simulink model "Buck_Boost_converter_Lab"  (R2020b)
settings: Solver=ode23tb  StartTime=0.0  StopTime=1  RelTol=1e-3
values from neighbouring files (symbols this model uses):
  C = 2200e-6    (= 0.0022)    [Parameters.m]    (also in Parameters_Buck_Boost.m = 0.00022; boost.m = 0.00022)
  d = 0.5    [Parameters.m]    (also in Parameters_Buck_Boost.m; boost.m)
  f = 5000    [Parameters.m]    (also in Parameters_Buck_Boost.m; boost.m)
  L = 820e-6    (= 0.00082)    [Parameters.m]    (also in Parameters_Buck_Boost.m = 0.0008; boost.m = 0.0008)
  R = 50    [Parameters.m]    (also in Parameters_Buck_Boost.m = 7; boost.m = 7)
  Vin = 5    [Parameters.m]    (also in Parameters_Buck_Boost.m = 14; boost.m = 14)
libraries: powerlib x21, powerlib_meascontrol x4
settings Model: Creator=ashka  LastModifiedBy=ashka

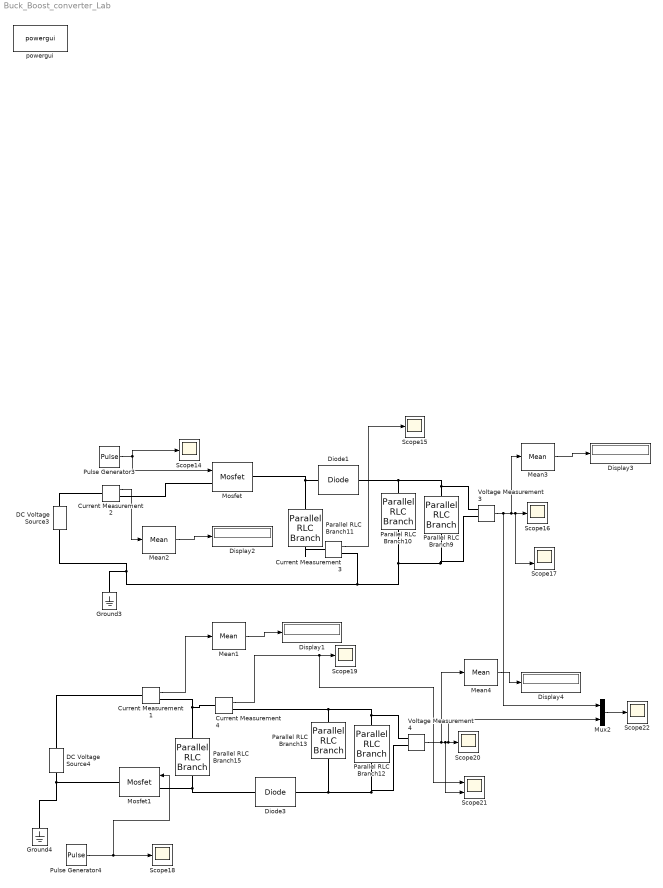
== system Buck_Boost_converter_Lab ==
  Current Measurement{1..4} (4 alike) : powerlib/Measurements/Current Measurement  PhasorSimulation=off  OutputType=Complex  PSBequivalent=0
  DC Voltage Source3 : powerlib/Electrical Sources/DC Voltage Source  Amplitude=Vin  Measurements=None
  DC Voltage Source4 : powerlib/Electrical Sources/DC Voltage Source  Amplitude=Vin  Measurements=None
  Diode1 : powerlib/Power Electronics/Diode  Ron=0.001  Lon=0  Vf=0.8  IC=0  UseSnubber=0  Rs=500  Cs=250e-9  Measurements=off
  Diode3 : powerlib/Power Electronics/Diode  Ron=0.001  Lon=0  Vf=0.8  IC=0  UseSnubber=0  Rs=500  Cs=250e-9  Measurements=off
  Display{1..4} (4 alike) : Display
  Ground3 : powerlib/Elements/Ground  LConnTagsString=a
  Ground4 : powerlib/Elements/Ground  LConnTagsString=a
  Mean1 : powerlib_meascontrol/Measurements/Mean  Freq=f  Vinit=0  Ts=0
  Mean2 : powerlib_meascontrol/Measurements/Mean  Freq=f  Vinit=0  Ts=0
  Mean3 : powerlib_meascontrol/Measurements/Mean  Freq=f  Vinit=0  Ts=0
  Mean4 : powerlib_meascontrol/Measurements/Mean  Freq=f  Vinit=7  Ts=0
  Mosfet : powerlib/Power Electronics/Mosfet  Ron=0.1  Lon=0  Rd=0.01  Vfd=0  IC=0  Rs=1e5  Cs=inf  Measurements=off
  Mosfet1 : powerlib/Power Electronics/Mosfet  Ron=0.1  Lon=0  Rd=0.01  Vfd=0  IC=0  Rs=1e5  Cs=inf  Measurements=off
  Mux2 : Mux  Inputs=2
  Parallel RLC Branch10 : powerlib/Elements/Parallel RLC Branch  LConnTagsString=a  RConnTagsString=__new0  BranchType=C  Resistance=10  Inductance=1e-3  SetiL0=off  InitialCurrent=0  Capacitance=C  Setx0=off  InitialVoltage=0  Measurements=None
  Parallel RLC Branch11 : powerlib/Elements/Parallel RLC Branch  LConnTagsString=a  RConnTagsString=__new0  BranchType=L  Resistance=10  Inductance=L  SetiL0=off  InitialCurrent=0  Capacitance=1e-6  Setx0=off  InitialVoltage=0  Measurements=None
  Parallel RLC Branch12 : powerlib/Elements/Parallel RLC Branch  LConnTagsString=a  RConnTagsString=__new0  BranchType=R  Resistance=R  Inductance=10e-3  SetiL0=off  InitialCurrent=0  Capacitance=1e-6  Setx0=off  InitialVoltage=0  Measurements=None
  Parallel RLC Branch13 : powerlib/Elements/Parallel RLC Branch  LConnTagsString=a  RConnTagsString=__new0  BranchType=C  Resistance=10  Inductance=1e-3  SetiL0=off  InitialCurrent=0  Capacitance=C  Setx0=off  InitialVoltage=0  Measurements=None
  Parallel RLC Branch15 : powerlib/Elements/Parallel RLC Branch  LConnTagsString=a  RConnTagsString=__new0  BranchType=L  Resistance=10  Inductance=L  SetiL0=off  InitialCurrent=0  Capacitance=1e-6  Setx0=off  InitialVoltage=0  Measurements=None
  Parallel RLC Branch9 : powerlib/Elements/Parallel RLC Branch  LConnTagsString=a  RConnTagsString=__new0  BranchType=R  Resistance=R  Inductance=10e-3  SetiL0=off  InitialCurrent=0  Capacitance=1e-6  Setx0=off  InitialVoltage=0  Measurements=None
  Pulse Generator3 : DiscretePulseGenerator  PulseType=Time based  Amplitude=10  Period=1/f  PulseWidth=d*100
  Pulse Generator4 : DiscretePulseGenerator  PulseType=Time based  Amplitude=10  Period=1/f  PulseWidth=d*100
  Scope{14..16,18..20,22} (7 alike) : Scope
  Scope17 : Scope  NumInputPorts=2
  Scope21 : Scope  NumInputPorts=2
  Voltage Measurement3 : powerlib/Measurements/Voltage Measurement  PhasorSimulation=off  OutputType=Complex  PSBequivalent=0
  Voltage Measurement4 : powerlib/Measurements/Voltage Measurement  PhasorSimulation=off  OutputType=Complex  PSBequivalent=0
  powergui : powerlib/powergui  Priority=1  SimulationMode=Continuous  SampleTime=50e-6  frequency=60  Iterations=50  frequencyindice=0  Pbase=100e6  ErrMax=1e-4  UnitsV=kV  UnitsW=MW  buscounter=0  FunctionMessages=off  echomessages=off  EnableUseOfTLC=off  CurrentSourceSwitches=off  DisableSnubberDevices=off  DisableRonSwitches=off  DisableVfSwitches=off  DisplayEquations=off  AutomaticDiscreteSolvers=off  SolverType=Tustin/Backward Euler (TBE)  Interpol=off  ExternalGateDelay=off  methode=off  Ts=100  x0status=blocks  SPID=on  SwTol=0  HookPort=off  NonlinearTolerance=1e-4  nMaxIteration=100  ContinueOnMaxIteration=off  RestoreLinks=warning  ResistiveCurrentMeasurement=off  Frange=[0:2:500]  Ylog=off  Xlog=on  ShowGrid=off  save=off  variable=ZData  structure=0  ZoomFFT=off  StartTime=0.0  cycles=1  DisplayStyle=1  fundamental=60  FreqAxis=off  MaxFrequency=1000  frequencyindicesteady=1  RmsSteady=1  display=off
  wires:
  Voltage Measurement3/1 -> Mux2/1, Scope17/2, Scope16/1, Mean3/1
  Current Measurement3/1 -> Scope15/1
  Mean3/1 -> Display3/1
  Pulse Generator3/1 -> Mosfet/1, Scope14/1
  Mux2/1 -> Scope22/1
  Current Measurement4/1 -> Scope21/1, Scope19/1
  Voltage Measurement4/1 -> Scope21/2, Mux2/2, Scope20/1, Mean4/1
  Mean4/1 -> Display4/1
  Pulse Generator4/1 -> Mosfet1/1, Scope18/1
  Mean1/1 -> Display1/1
  Current Measurement1/1 -> Mean1/1
  Mean2/1 -> Display2/1
  Current Measurement2/1 -> Mean2/1
  connections:
  Parallel RLC Branch11/LConn1 -- Current Measurement3/LConn1
  Parallel RLC Branch10/LConn1 -- Diode1/LConn1 -- Voltage Measurement3/LConn1 -- Parallel RLC Branch9/LConn1
  Parallel RLC Branch11/RConn1 -- Diode1/RConn1 -- Mosfet/RConn1
  Ground3/LConn1 -- Current Measurement3/RConn1 -- Parallel RLC Branch10/RConn1 -- Voltage Measurement3/LConn2 -- Parallel RLC Branch9/RConn1 -- DC Voltage Source3/LConn1
  DC Voltage Source4/LConn1 -- Mosfet1/RConn1 -- Ground4/LConn1
  Parallel RLC Branch13/RConn1 -- Diode3/RConn1 -- Voltage Measurement4/LConn2 -- Parallel RLC Branch12/RConn1
  Parallel RLC Branch13/LConn1 -- Current Measurement4/RConn1 -- Parallel RLC Branch12/LConn1 -- Voltage Measurement4/LConn1
  Parallel RLC Branch15/LConn1 -- Diode3/LConn1 -- Mosfet1/LConn1
  DC Voltage Source4/RConn1 -- Current Measurement1/LConn1
  Current Measurement1/RConn1 -- Current Measurement4/LConn1 -- Parallel RLC Branch15/RConn1
  Current Measurement2/LConn1 -- DC Voltage Source3/RConn1
  Current Measurement2/RConn1 -- Mosfet/LConn1
